simulink model "kinematic_vehicle_demo"  (R2019b)
settings: Solver=FixedStepDiscrete  StartTime=0.0  StopTime=40  FixedStep=0.01  RelTol=1e-3  EnableMultiTasking=on
libraries: simulink x2
Description:
  | Counter Implemented in a C++ S-function
settings Model: ExtModeTrigMode=oneshot  ExtModeArmWhenConnect=off  ExtModeAutoUpdateStatusClock=off  Creator=The MathWorks, Inc.  LastModifiedBy=chr
settings DataIOCC: SaveFormat=Array
settings OptimizationCC: BlockReduction=off  BooleanDataType=off  ExpressionDepthLimit=2147483647  InitFltsAndDblsToZero=on  LifeSpan=inf
settings DebuggingCC: SaveWithParameterizedLinksMsg=none  SignalResolutionControl=TryResolveAllWithWarning  MultiTaskDSMMsg=warning  MultiTaskCondExecSysMsg=none  FcnCallInpInsideContextMsg=warning  StateNameClashWarn=warning  SFUnexpectedBacktrackingDiag=warning  SFNoUnconditionalDefaultTransitionDiag=warning  SFExecutionAtInitializationDiag=none  ArithmeticOperatorsInVariantConditions=warning
settings HardwareCC: ProdBitPerPointer=32  ProdBitPerSizeT=32  ProdBitPerPtrDiffT=32  ProdLargestAtomicFloat=None  ProdIntDivRoundTo=Undefined  ProdEndianess=Unspecified  ProdWordSize=32  ProdHWDeviceType=32-bit Generic
settings ModelReferenceCC: PropagateSignalLabelsOutOfModel=off
settings SFSimCC: SimUseLocalCustomCode=off  CustomCodeUndefinedFunction=UseInterfaceOnly
settings RTWCC: Description=Generic Real-Time Target  RetainRTWFile=on  RTWUseLocalCustomCode=off
settings CodeAppCC: StateflowObjectComments=on
settings GRTTargetCC: TargetFcnLib=ansi_tfl_tmw.mat  TargetLangStandard=C89/C90 (ANSI)  GeneratePreprocessorConditionals=Disable all  CombineOutputUpdateFcns=off  GRTInterface=on
settings ConfigComp: CovMetricSettings=dw  CovHtmlReporting=on  CovSaveCumulativeToWorkspaceVar=on  CovSaveSingleToWorkspaceVar=on  CovExternalEMLEnable=off

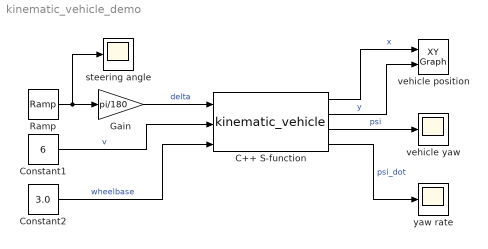
== system kinematic_vehicle_demo ==
  C++ S-function : S-Function  FunctionName=kinematic_vehicle  Parameters=0  SFunctionDeploymentMode=off  EnableBusSupport=off
  Constant1 : Constant  Value=6
  Constant2 : Constant  Value=3.0
  Gain : Gain  Gain=pi/180
  Ramp : simulink/Sources/Ramp  slope=-0.5  start=0  InitialOutput=20
  steering angle : Scope
  vehicle position : simulink/Sinks/XY Graph  xmin=-40  xmax=40  ymin=-40  ymax=40  st=-1
  vehicle yaw : Scope
  yaw rate : Scope
  wires:
  Constant2/1 -> C++ S-function/3  "wheelbase"
  Ramp/1 -> steering angle/1, Gain/1
  Gain/1 -> C++ S-function/1  "delta"
  Constant1/1 -> C++ S-function/2  "v"
  C++ S-function/1 -> vehicle position/1  "x"
  C++ S-function/2 -> vehicle position/2  "y"
  C++ S-function/3 -> vehicle yaw/1  "psi"
  C++ S-function/4 -> yaw rate/1  "psi_dot"
